simulink subsystem "rss_SplyVltgHiLvl1Dia"  (R2023a)
settings: Solver=VariableStepAuto  StartTime=0.0  StopTime=10.0  RelTol=1e-3
undefined symbols (not defined in the file): Cdbl_uSplyVltgMaxVal, ENM_TYPE_FALT, Gu16_ctSplyVltgHiLvl1ConfCnt_C, Gu16_ctSplyVltgHiLvl1RcvyCnt_C, Gu16_uSplyVltgHiLvl1ConfTrs_C, Gu16_uSplyVltgHiLvl1RcvyTrs_C
libraries: vhit_control_library x1, lib_fault_definiteness x1
settings Model: Creator=xiaoqiang.yuan  LastModifiedBy=xiaoqiang.yuan

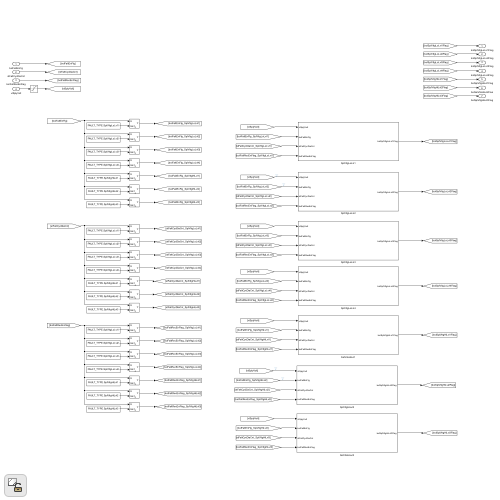
[thumbnail: Simulink's stored preview of the top-level diagram]
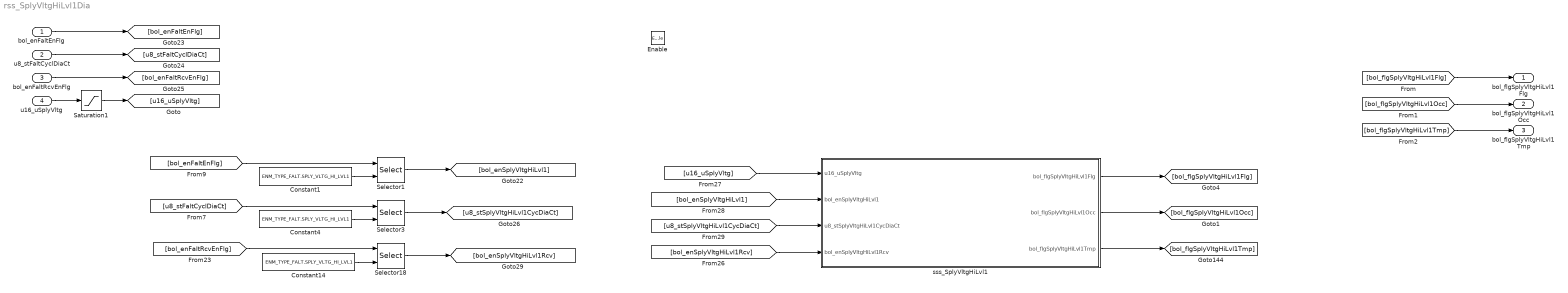
== system rss_SplyVltgHiLvl1Dia ==
  bol_enFaltEnFlg : Inport  OutDataTypeStr=boolean
  u8_stFaltCyclDiaCt : Inport  Port=2  OutDataTypeStr=uint8
  bol_enFaltRcvEnFlg : Inport  Port=3  OutDataTypeStr=boolean
  u16_uSplyVltg : Inport  Port=4  OutDataTypeStr=dt_Standardize_u16p15b0
  Enable : EnablePort
  Constant1 : Constant  Value=ENM_TYPE_FALT.SPLY_VLTG_HI_LVL1
  Constant14 : Constant  Value=ENM_TYPE_FALT.SPLY_VLTG_HI_LVL1
  Constant4 : Constant  Value=ENM_TYPE_FALT.SPLY_VLTG_HI_LVL1
  Saturation1 : Saturate  UpperLimit=Cdbl_uSplyVltgMaxVal  LowerLimit=0
  Selector1 : Selector  IndexMode=Zero-based  InputPortWidth=Cdbl_numFaltDiaNum  IndexOptions=Index vector (port)  Indices=[1 3]  OutputSizes=1
  Selector18 : Selector  IndexMode=Zero-based  InputPortWidth=Cdbl_numFaltDiaNum  IndexOptions=Index vector (port)  Indices=[1 3]  OutputSizes=1
  Selector3 : Selector  IndexMode=Zero-based  InputPortWidth=Cdbl_numFaltDiaNum  IndexOptions=Index vector (port)  Indices=[1 3]  OutputSizes=1
  sss_SplyVltgHiLvl1 : Subsystem
  bol_flgSplyVltgHiLvl1Flg : Outport  OutDataTypeStr=boolean
  bol_flgSplyVltgHiLvl1Occ : Outport  Port=2  OutDataTypeStr=boolean
  bol_flgSplyVltgHiLvl1Tmp : Outport  Port=3  OutDataTypeStr=boolean
  wires:
  [bol_flgSplyVltgHiLvl1Flg] -> bol_flgSplyVltgHiLvl1Flg/1
  Constant1/1 -> Selector1/2
  [bol_enFaltEnFlg] -> Selector1/1
  Selector1/1 -> [bol_enSplyVltgHiLvl1]
  bol_enFaltEnFlg/1 -> [bol_enFaltEnFlg]
  bol_enFaltRcvEnFlg/1 -> [bol_enFaltRcvEnFlg]
  u8_stFaltCyclDiaCt/1 -> [u8_stFaltCyclDiaCt]
  Selector3/1 -> [u8_stSplyVltgHiLvl1CycDiaCt]
  [u8_stFaltCyclDiaCt] -> Selector3/1
  Selector18/1 -> [bol_enSplyVltgHiLvl1Rcv]
  [bol_enSplyVltgHiLvl1] -> sss_SplyVltgHiLvl1/2(bol_enSplyVltgHiLvl1)
  sss_SplyVltgHiLvl1/1(bol_flgSplyVltgHiLvl1Flg) -> [bol_flgSplyVltgHiLvl1Flg]
  [bol_enSplyVltgHiLvl1Rcv] -> sss_SplyVltgHiLvl1/4(bol_enSplyVltgHiLvl1Rcv)
  [u8_stSplyVltgHiLvl1CycDiaCt] -> sss_SplyVltgHiLvl1/3(u8_stSplyVltgHiLvl1CycDiaCt)
  [u16_uSplyVltg] -> sss_SplyVltgHiLvl1/1(u16_uSplyVltg)
  u16_uSplyVltg/1 -> Saturation1/1
  Saturation1/1 -> [u16_uSplyVltg]
  Constant4/1 -> Selector3/2
  [bol_enFaltRcvEnFlg] -> Selector18/1
  Constant14/1 -> Selector18/2
  sss_SplyVltgHiLvl1/2(bol_flgSplyVltgHiLvl1Occ) -> [bol_flgSplyVltgHiLvl1Occ]
  [bol_flgSplyVltgHiLvl1Occ] -> bol_flgSplyVltgHiLvl1Occ/1
  [bol_flgSplyVltgHiLvl1Tmp] -> bol_flgSplyVltgHiLvl1Tmp/1
  sss_SplyVltgHiLvl1/3(bol_flgSplyVltgHiLvl1Tmp) -> [bol_flgSplyVltgHiLvl1Tmp]

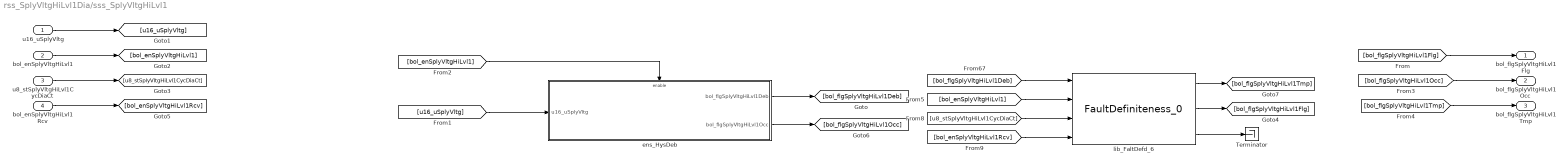
== system rss_SplyVltgHiLvl1Dia/sss_SplyVltgHiLvl1 ==
  u16_uSplyVltg : Inport
  bol_enSplyVltgHiLvl1 : Inport  Port=2
  u8_stSplyVltgHiLvl1CycDiaCt : Inport  Port=3
  bol_enSplyVltgHiLvl1Rcv : Inport  Port=4
  Terminator : Terminator
  ens_HysDeb : Subsystem
  lib_FaltDefd_6 : lib_fault_definiteness/FaultDefiniteness_0  lb_FaltWaitRecvCnt=Gu16_ctSplyVltgHiLvl1ConfCnt_C
  bol_flgSplyVltgHiLvl1Flg : Outport
  bol_flgSplyVltgHiLvl1Occ : Outport  Port=2
  bol_flgSplyVltgHiLvl1Tmp : Outport  Port=3
  wires:
  [bol_flgSplyVltgHiLvl1Tmp] -> bol_flgSplyVltgHiLvl1Tmp/1
  [bol_flgSplyVltgHiLvl1Occ] -> bol_flgSplyVltgHiLvl1Occ/1
  ens_HysDeb/2(bol_flgSplyVltgHiLvl1Occ) -> [bol_flgSplyVltgHiLvl1Occ]
  lib_FaltDefd_6/1 -> [bol_flgSplyVltgHiLvl1Tmp]
  lib_FaltDefd_6/2 -> [bol_flgSplyVltgHiLvl1Flg]
  lib_FaltDefd_6/3 -> Terminator/1
  [bol_enSplyVltgHiLvl1] -> ens_HysDeb/Enable
  [u16_uSplyVltg] -> ens_HysDeb/1(u16_uSplyVltg)
  ens_HysDeb/1(bol_flgSplyVltgHiLvl1Deb) -> [bol_flgSplyVltgHiLvl1Deb]
  bol_enSplyVltgHiLvl1Rcv/1 -> [bol_enSplyVltgHiLvl1Rcv]
  u8_stSplyVltgHiLvl1CycDiaCt/1 -> [u8_stSplyVltgHiLvl1CycDiaCt]
  bol_enSplyVltgHiLvl1/1 -> [bol_enSplyVltgHiLvl1]
  [bol_flgSplyVltgHiLvl1Flg] -> bol_flgSplyVltgHiLvl1Flg/1
  u16_uSplyVltg/1 -> [u16_uSplyVltg]
  [bol_enSplyVltgHiLvl1Rcv] -> lib_FaltDefd_6/4
  [u8_stSplyVltgHiLvl1CycDiaCt] -> lib_FaltDefd_6/3
  [bol_enSplyVltgHiLvl1] -> lib_FaltDefd_6/2
  [bol_flgSplyVltgHiLvl1Deb] -> lib_FaltDefd_6/1

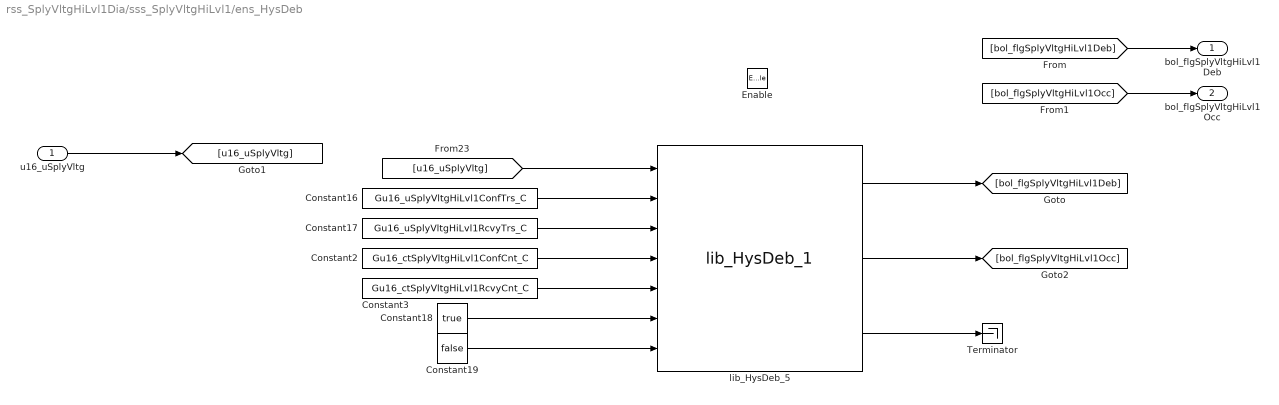
== system rss_SplyVltgHiLvl1Dia/sss_SplyVltgHiLvl1/ens_HysDeb ==
  u16_uSplyVltg : Inport
  Enable : EnablePort
  Constant16 : Constant  Value=Gu16_uSplyVltgHiLvl1ConfTrs_C
  Constant17 : Constant  Value=Gu16_uSplyVltgHiLvl1RcvyTrs_C
  Constant18 : Constant  Value=true  OutDataTypeStr=boolean
  Constant19 : Constant  Value=false  OutDataTypeStr=boolean
  Constant2 : Constant  Value=Gu16_ctSplyVltgHiLvl1ConfCnt_C
  Constant3 : Constant  Value=Gu16_ctSplyVltgHiLvl1RcvyCnt_C
  Terminator : Terminator
  lib_HysDeb_5 : vhit_control_library/lib_HysDeb_1  lb_parInitOutp=0
  bol_flgSplyVltgHiLvl1Deb : Outport
  bol_flgSplyVltgHiLvl1Occ : Outport  Port=2
  wires:
  lib_HysDeb_5/3 -> Terminator/1
  [bol_flgSplyVltgHiLvl1Occ] -> bol_flgSplyVltgHiLvl1Occ/1
  lib_HysDeb_5/2 -> [bol_flgSplyVltgHiLvl1Occ]
  Constant3/1 -> lib_HysDeb_5/5
  Constant2/1 -> lib_HysDeb_5/4
  Constant19/1 -> lib_HysDeb_5/7
  Constant18/1 -> lib_HysDeb_5/6
  Constant17/1 -> lib_HysDeb_5/3
  Constant16/1 -> lib_HysDeb_5/2
  [u16_uSplyVltg] -> lib_HysDeb_5/1
  u16_uSplyVltg/1 -> [u16_uSplyVltg]
  [bol_flgSplyVltgHiLvl1Deb] -> bol_flgSplyVltgHiLvl1Deb/1
  lib_HysDeb_5/1 -> [bol_flgSplyVltgHiLvl1Deb]
